simulink library "lib_Convection_LamFlatPlate_ChurchillOzoe"  (R2015a)
settings: Solver=ode45  StartTime=0.0  StopTime=10.0  RelTol=1e-3
libraries: simulink x1
settings Model: Creator=jlkratz  LastModifiedBy=jlkratz

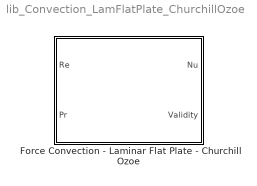
== system lib_Convection_LamFlatPlate_ChurchillOzoe ==
  Force Convection - Laminar Flat Plate - Churchill Ozoe : Subsystem  mask(TSAT: Laminar Flat Plate - Churchill Ozoe){LocalOrAvg_M=Average Nusselt number}
      mask help:
      | This block estimates the Nusselt number of an external flow over an isothermal laminar flat plate using a correlation developed by Churchill and Ozoe. This single correlation is valid for all Prandtl numbers. It can either calculate the local or average Nusselt number over 1 surface of the plate. If the average Nusselt number is to be calcualted then assure the charateristic length used to calculate the Reynolds Number is the full length of the plate. Note that all fluid properrties should be evaluated at film temperature (average of the bulk fluid and surface temperatures). Beyond the flow being laminar the implemented correlations also requires:
      |
      | Pe >= 100 (Peclet number, Pe = Re*Pr)
      |
      | If this contraint is not met then the "Validity" output will be 1, and otherwise will be 0. For more information on the implemented correlations and function of the block, see the block help menu.
      mask Help: web(which('Convection_TSAT_LaminarFlatPlate_ChurchillOzoe.html'),'-helpbrowser')
      mask TypeOptions LocalOrAvg_M: Local Nusselt number | Average Nusselt number

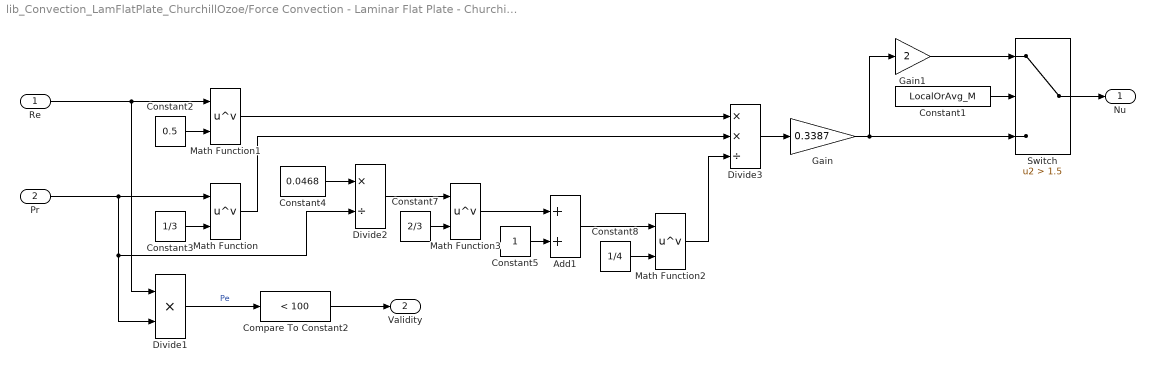
== system lib_Convection_LamFlatPlate_ChurchillOzoe/Force Convection - Laminar Flat Plate - Churchill Ozoe ==
  Re : Inport
  Pr : Inport  Port=2
  Add1 : Sum
  Compare To Constant2 : simulink/Logic and Bit Operations/Compare To Constant  relop=<  const=100  OutDataTypeStr=boolean
  Constant1 : Constant  Value=LocalOrAvg_M
  Constant2 : Constant  Value=0.5
  Constant3 : Constant  Value=1/3
  Constant4 : Constant  Value=0.0468
  Constant5 : Constant
  Constant7 : Constant  Value=2/3
  Constant8 : Constant  Value=1/4
  Divide1 : Product  Inputs=**
  Divide2 : Product  Inputs=*/
  Divide3 : Product  Inputs=**/
  Gain : Gain  Gain=0.3387
  Gain1 : Gain  Gain=2
  Math Function{,1..3} (4 alike) : Math  Operator=pow  SaturateOnIntegerOverflow=on
  Switch : Switch  Criteria=u2 > Threshold  Threshold=1.5
  Nu : Outport
  Validity : Outport  Port=2
  wires:
  Constant1/1 -> Switch/2
  Switch/1 -> Nu/1
  Gain1/1 -> Switch/1
  Gain/1 -> Gain1/1, Switch/3
  Math Function1/1 -> Divide3/1
  Pr/1 -> Divide1/2, Divide2/2, Math Function/1
  Re/1 -> Math Function1/1, Divide1/1
  Constant8/1 -> Math Function2/2
  Add1/1 -> Math Function2/1
  Constant2/1 -> Math Function1/2
  Divide2/1 -> Math Function3/1
  Constant3/1 -> Math Function/2
  Math Function2/1 -> Divide3/3
  Math Function/1 -> Divide3/2
  Divide1/1 -> Compare To Constant2/1  "Pe"
  Compare To Constant2/1 -> Validity/1
  Constant4/1 -> Divide2/1
  Divide3/1 -> Gain/1
  Math Function3/1 -> Add1/1
  Constant7/1 -> Math Function3/2
  Constant5/1 -> Add1/2
